simulink model "cubesat_propagation"  (R2019b)
settings: Solver=FixedStepAuto  StartTime=0.0  StopTime=5  FixedStep=dT  RelTol=1e-5
PostLoadFcn:
  | if builtin('license','test','Virtual_Reality_Toolbox')
  |     set_param([bdroot(gcs) '/Simulink 3D Animation'], 'enableVis', 'on')
  | else
  |     set_param([bdroot(gcs) '/Simulink 3D Animation'], 'enableVis', 'off')
  | end
InitFcn:
  | if strcmp(get_param([bdroot(gcs) '/Simulink 3D Animation'], 'enableVis'), 'on')
  |     if ~builtin('license','checkout','Virtual_Reality_Toolbox')
  |         error(message('aeroblks_cubesat:cubesat:licenseFailAnimTemplate'));
  |     end
  | end
model workspace (MATLAB code in the model file + MAT data in the model file):
  aeroCoeff.Cl0 = 0.000591
  aeroCoeff.Cl_beta = -0.0618
  aeroCoeff.Cl_da = -0.09917
  aeroCoeff.Cl_da_alpha = -0.08269
  aeroCoeff.Cl_dr = 0.006934
  aeroCoeff.Cl_p = -0.5045
  aeroCoeff.Cl_r = 0.1695
  aeroCoeff.Cm0 = 0.09448
  aeroCoeff.Cm_alpha = -0.6028
  aeroCoeff.Cm_alpha2 = -2.14
  aeroCoeff.Cm_beta2 = 0.6921
  aeroCoeff.Cm_de = -1.921
  aeroCoeff.Cm_df = 0.4072
  aeroCoeff.Cm_q = -15.56
  aeroCoeff.Cm_r = -0.3118
  aeroCoeff.Cn0 = -0.003117
  aeroCoeff.Cn_beta = 0.006719
  aeroCoeff.Cn_beta3 = 0.1373
  aeroCoeff.Cn_da = -0.003872
  aeroCoeff.Cn_dr = -0.08265
  aeroCoeff.Cn_p = -0.1585
  aeroCoeff.Cn_q = 0.1595
  aeroCoeff.Cn_r = -0.1112
  aeroCoeff.Cx0 = -0.03554
  aeroCoeff.Cx_alpha = 0.00292
  aeroCoeff.Cx_alpha2 = 5.459
  aeroCoeff.Cx_alpha3 = -5.162
  aeroCoeff.Cx_df = -0.09447
  aeroCoeff.Cx_df_alpha = 1.106
  aeroCoeff.Cx_dr = 0.03412
  aeroCoeff.Cx_q = -0.6748
  aeroCoeff.Cy0 = -0.002226
  aeroCoeff.Cy_beta = -0.7678
  aeroCoeff.Cy_da = -0.02956
  aeroCoeff.Cy_dr = 0.1158
  aeroCoeff.Cy_dr_alpha = 0.5238
  aeroCoeff.Cy_p = -0.124
  aeroCoeff.Cy_r = 0.3666
  aeroCoeff.Cz0 = -0.05504
  aeroCoeff.Cz_alpha = -5.578
  aeroCoeff.Cz_alpha3 = 3.442
  aeroCoeff.Cz_de = -0.398
  aeroCoeff.Cz_de_beta = -15.93
  aeroCoeff.Cz_df = -1.377
  aeroCoeff.Cz_df_alpha = -1.261
  aeroCoeff.Cz_q = -2.988
  environment.EarthRefAlt = 0
  initCond.x0 = [0 0 -2202]
  initCond.v0 = [44.54 2.714 5.836]
  initCond.euler0 = [0 0.1308996939 0]
  initCond.w0 = [0 0 0]
  inputs0.time = 0
  inputs0.signals(1).dimensions = 1
  inputs0.signals(1).values = -0.104711430294
  inputs0.signals(2).dimensions = 1
  inputs0.signals(2).values = -0.0698725229544
  inputs0.signals(3).dimensions = 1
  inputs0.signals(3).values = -0.000215042330254
  states0.time = 0
  states0.signals(1).values = [0 0 -2202]
  states0.signals(1).dimensions = 3
  states0.signals(1).label = 'CSTATE'
  states0.signals(1).blockName = 'asb6DOFAirframeTemplate/6DOF EOM/6DOF (Euler Angles)/xe,ye,ze'
  states0.signals(1).stateName = ''
  states0.signals(1).inReferencedModel = 0
  states0.signals(1).sampleTime = [0 0]
  states0.signals(2).values = [0.128665353089 0.259337659946 -0.178947917154]
  states0.signals(2).dimensions = 3
  states0.signals(2).label = 'CSTATE'
  states0.signals(2).blockName = 'asb6DOFAirframeTemplate/6DOF EOM/6DOF (Euler Angles)/Calculate DCM &
    | Euler Angles/phi
    | theta
    | psi'
  states0.signals(2).stateName = ''
  states0.signals(2).inReferencedModel = 0
  states0.signals(2).sampleTime = [0 0]
  states0.signals(3).values = [36.9119692666 8.10720863264 8.82591882596]
  states0.signals(3).dimensions = 3
  states0.signals(3).label = 'CSTATE'
  states0.signals(3).blockName = 'asb6DOFAirframeTemplate/6DOF EOM/6DOF (Euler Angles)/ub,vb,wb'
  states0.signals(3).stateName = ''
  states0.signals(3).inReferencedModel = 0
  states0.signals(3).sampleTime = [0 0]
  states0.signals(4).values = [0 0 0]
  states0.signals(4).dimensions = 3
  states0.signals(4).label = 'CSTATE'
  states0.signals(4).blockName = 'asb6DOFAirframeTemplate/6DOF EOM/6DOF (Euler Angles)/p,q,r '
  states0.signals(4).stateName = ''
  states0.signals(4).inReferencedModel = 0
  states0.signals(4).sampleTime = [0 0]
  states0.signals(5).values = [0 0]
  states0.signals(5).dimensions = 2
  states0.signals(5).label = 'CSTATE'
  states0.signals(5).blockName = 'asb6DOFAirframeTemplate/Environment Model/Dryden Wind Turbulence Model 
    | (Continuous (+q +r))/Filters on velocities/Hwgw(s)/wg_p1'
  states0.signals(5).stateName = ''
  states0.signals(5).inReferencedModel = 0
  states0.signals(5).sampleTime = [0 0]
  states0.signals(6).values = [0 0]
  states0.signals(6).dimensions = 2
  states0.signals(6).label = 'CSTATE'
  states0.signals(6).blockName = 'asb6DOFAirframeTemplate/Environment Model/Dryden Wind Turbulence Model 
    | (Continuous (+q +r))/Filters on velocities/Hwgw(s)/wg_p2'
  states0.signals(6).stateName = ''
  states0.signals(6).inReferencedModel = 0
  states0.signals(6).sampleTime = [0 0]
  states0.signals(7).values = [0 0]
  states0.signals(7).dimensions = 2
  states0.signals(7).label = 'CSTATE'
  states0.signals(7).blockName = 'asb6DOFAirframeTemplate/Environment Model/Dryden Wind Turbulence Model 
    | (Continuous (+q +r))/Filters on velocities/Hvgw(s)/vg_p1'
  states0.signals(7).stateName = ''
  states0.signals(7).inReferencedModel = 0
  states0.signals(7).sampleTime = [0 0]
  states0.signals(8).values = [0 0]
  states0.signals(8).dimensions = 2
  states0.signals(8).label = 'CSTATE'
  states0.signals(8).blockName = 'asb6DOFAirframeTemplate/Environment Model/Dryden Wind Turbulence Model 
    | (Continuous (+q +r))/Filters on velocities/Hvgw(s)/vgw_p2'
  states0.signals(8).stateName = ''
  states0.signals(8).inReferencedModel = 0
  states0.signals(8).sampleTime = [0 0]
  states0.signals(9).values = [0 0]
  states0.signals(9).dimensions = 2
  states0.signals(9).label = 'CSTATE'
  states0.signals(9).blockName = 'asb6DOFAirframeTemplate/Environment Model/Dryden Wind Turbulence Model 
    | (Continuous (+q +r))/Filters on velocities/Hugw(s)/ug_p'
  states0.signals(9).stateName = ''
  states0.signals(9).inReferencedModel = 0
  states0.signals(9).sampleTime = [0 0]
  states0.signals(10).values = [0 0]
  states0.signals(10).dimensions = 2
  states0.signals(10).label = 'CSTATE'
  states0.signals(10).blockName = 'asb6DOFAirframeTemplate/Environment Model/Dryden Wind Turbulence Model 
    | (Continuous (+q +r))/Filters on angular rates/Hrgw/rgw_p'
  states0.signals(10).stateName = ''
  states0.signals(10).inReferencedModel = 0
  states0.signals(10).sampleTime = [0 0]
  states0.signals(11).values = [0 0]
  states0.signals(11).dimensions = 2
  states0.signals(11).label = 'CSTATE'
  states0.signals(11).blockName = 'asb6DOFAirframeTemplate/Environment Model/Dryden Wind Turbulence Model 
    | (Continuous (+q +r))/Filters on angular rates/Hqgw/qgw_p'
  states0.signals(11).stateName = ''
  states0.signals(11).inReferencedModel = 0
  states0.signals(11).sampleTime = [0 0]
  states0.signals(12).values = [0 0]
  states0.signals(12).dimensions = 2
  states0.signals(12).label = 'CSTATE'
  states0.signals(12).blockName = 'asb6DOFAirframeTemplate/Environment Model/Dryden Wind Turbulence Model 
    | (Continuous (+q +r))/Filters on angular rates/Hpgw/pgw_p'
  states0.signals(12).stateName = ''
  states0.signals(12).inReferencedModel = 0
  states0.signals(12).sampleTime = [0 0]
  vehicle.Sref = 23.23
  vehicle.cbar = 1.5875
  vehicle.bref = 14.63
  vehicle.CG = [0 0 0]
  vehicle.CP = [0 0 0]
  vehicle.inertia = [5788  0  117.6; 0  6928.9  0; -117.6  0  11578.3]
  vehicle.acMass = 2288.231
  vehicle.Thrust = 2300
  vehicle.aileron_max = 0.523598775598
  vehicle.aileron_min = -0.523598775598
  vehicle.elevator_max = 0.523598775598
  vehicle.elevator_min = -0.523598775598
  vehicle.rudder_max = 1.0471975512
  vehicle.rudder_min = -1.0471975512
  other statements: initialize6DOFSkyHogg;
values from neighbouring files (symbols this model uses):
  a = (mu^(1/3))/((2*n*pi/86400)^(2/3))+0.01e5    (= 6961989.91401)    [pwsat2_setup.m]
  e = 0.0011871    [pwsat2_setup.m]
  incl = deg2rad(97.7672)    [pwsat2_setup.m]
  initEuler = [0 0 0]    [pwsat2_setup.m]
  julian = juliandate(utc)    [pwsat2_setup.m]
  RA = deg2rad(56.1804)    [pwsat2_setup.m]
  w = deg2rad(236.0402)    [pwsat2_setup.m]
undefined symbols (not defined in the file or in its folder): constraintAxes, Earth, euler0, km, pointing, pqr0, s, TA, WGS84
libraries: aerolibutil x13, aerolibconvert2 x5, sharedtransform x3, asbCubeSatBlockLib x2, simulink x2, aerolibcelestial x2, aerolib6dof2 x1, aerolibtransform2 x1, sharedutil x1, aerolibobsolete x1, vrlib x1, aerolibgravity2 x1
(part 1 of 2)
settings Model: Creator=asmialek  LastModifiedBy=asmialek
settings SolverCC: AutoInsertRateTranBlk=on  InsertRTBMode=Never (minimum delay)  MinimalZcImpactIntegration=on
settings DataIOCC: SaveFormat=Array  SaveOutput=off  SignalLogging=off  DSMLogging=off  ReturnWorkspaceOutputsName=cube
settings OptimizationCC: EnhancedBackFolding=on  StrengthReduction=on  InitFltsAndDblsToZero=on  DifferentSizesBufferReuse=on
settings DebuggingCC: WriteAfterWriteMsg=DisableAll  AlgebraicLoopMsg=none  FcnCallInpInsideContextMsg=warning  UnconnectedInputMsg=none  UnconnectedOutputMsg=none  UnconnectedLineMsg=none  UniqueDataStoreMsg=error  RootOutportRequireBusObject=none  StateNameClashWarn=warning  PregeneratedLibrarySubsystemCodeDiagnostic=none  StrictBusMsg=ErrorOnBusTreatedAsVector  SFUnexpectedBacktrackingDiag=warning  SFNoUnconditionalDefaultTransitionDiag=warning  SFExecutionAtInitializationDiag=none  ArithmeticOperatorsInVariantConditions=warning
settings ModelReferenceCC: PropagateSignalLabelsOutOfModel=off
settings SFSimCC: SimUseLocalCustomCode=off  CustomCodeUndefinedFunction=UseInterfaceOnly
settings RTWCC: RTWUseLocalCustomCode=off
settings CodeAppCC: StateflowObjectComments=on

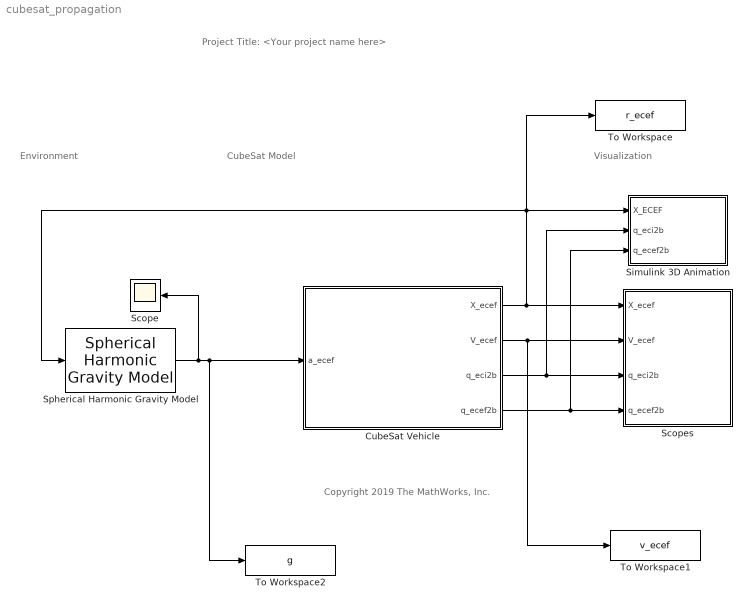
== system cubesat_propagation ==
  note: Project Title: <Your project name here>
  note: Copyright 2019 The MathWorks, Inc.
  note: Visualization
  note: Environment
  note: CubeSat Model
  CubeSat Vehicle : Subsystem  AncestorBlock=asbCubeSatBlockLib/CubeSat Vehicle  BlockKeywords=__PRM__SERIALIZED__DATA__:cube sat,cube sat vehicle,satellite,nanosat,nano sat,nanosatellite,nano satellite,pico sat,picosat,pico satellite,picosatellite,orbit propagator,orbit propagation,orbital propagator,orbital dynamics,astrodynamics,astro dynamics,spacecraft,space craft,space vehicle,spaceflight,space flight,low Earth orbit,low-Earth orbit,attitude control,kepler,keplerian elements,orbital elements,ECI,ECEF,Earth orientation parameters  mask(CubeSat Vehicle){sim_t0=julian, method=Keplerian Orbital Elements, epoch=2451545, a=a, ecc=e, incl=rad2deg(incl), omega=rad2deg(RA), argp=rad2deg(w), nu=rad2deg(TA), truelon=0, arglat=0, lonper=0, r_eci=[0 0 0], v_eci=[0 0 0], r_ecef=[0 0 0], v_ecef=[0 0 0], lla=[0 0 0], v_ned=[0 0 0], euler=initEuler, pqr=[0 0 0], pointingMode=Standby (Off), firstAlignExt=Dialog, firstAlign=[0 0 1], secondAlignExt=Dialog, secondAlign=[0 1 0], constraintCoord=ECI Axes, firstRefExt=Dialog, firstRef=[1 0 0], secondRefExt=Dialog, secondRef=[0 0 1], eopExt=Dialog, dAT=37, dUT1=-0.1193, pm=[0.2141e-4 0.6930e-4], dCIP=[0.1014e-6  -0.0681e-6], lod=0, missionRTSource=Dialog, missionRT=6*60*60, missionGS=[42, -71], missionTOICheck=on, missionTOI=[], missionEta=55, missionName=}
      mask prompts: sim_t0 "aeroblks_cubesat:cubesat:StartDate"; method "aeroblks_cubesat:cubesat:InputMethod"; epoch "aeroblks_cubesat:cubesat:ECIEpoch"; a "aeroblks_cubesat:cubesat:SemiMajorAxis"; ecc "aeroblks_cubesat:cubesat:Eccentricity"; incl "aeroblks_cubesat:cubesat:Inclination"; omega "aeroblks_cubesat:cubesat:RAAN"; argp "aeroblks_cubesat:cubesat:ArgP"; nu "aeroblks_cubesat:cubesat:TrueAnomaly"; truelon "aeroblks_cubesat:cubesat:TrueLon"; arglat "aeroblks_cubesat:cubesat:ArgLat"; lonper "aeroblks_cubesat:cubesat:LonPer"; r_eci "aeroblks_cubesat:cubesat:ECIPos"; v_eci "aeroblks_cubesat:cubesat:ECIVel"; r_ecef "aeroblks_cubesat:cubesat:ECEFPos"; v_ecef "aeroblks_cubesat:cubesat:ECEFVel"; lla "aeroblks_cubesat:cubesat:LLA"; v_ned "aeroblks_cubesat:cubesat:NEDVel"; euler "aeroblks_cubesat:cubesat:Euler"; pqr "aeroblks_cubesat:cubesat:BodyAngRates"; pointingMode "aeroblks_cubesat:cubesat:PointingMode"; constraintCoord "aeroblks_cubesat:cubesat:ConstaintCoord"; eopExt "aeroblks_cubesat:cubesat:EOPPulldown"; dAT "aeroblks_cubesat:cubesat:dTAI"; dUT1 "aeroblks_cubesat:cubesat:DUT1"; pm "aeroblks_cubesat:cubesat:DPolar"; dCIP "aeroblks_cubesat:cubesat:DCIP"; lod "aeroblks_cubesat:cubesat:DLOD"; missionRTSource "aeroblks_cubesat:cubesat:MissRunTimeSource"; missionRT "aeroblks_cubesat:cubesat:MissRunTime"; missionGS "aeroblks_cubesat:cubesat:MissGS"; missionTOICheck "aeroblks_cubesat:cubesat:MissTOICheckbox"; missionTOI "aeroblks_cubesat:cubesat:MissTOI"; missionEta "aeroblks_cubesat:cubesat:MissEta"; missionName "aeroblks_cubesat:cubesat:MissFileName"
      mask help: aeroblks_cubesat:cubesat:CubeSatBlockDesc
      mask init:
      | [lla0, uvw0, euler0, pqr0, thGAST0, ports, constraintAxes, pointing]  = cubesatBlockCallback(...
      |     gcb, 'init', method, sim_t0, epoch, a, ecc, incl, omega,...
      |     argp, nu, truelon, arglat, lonper,r_eci, v_eci, r_ecef, v_ecef,...
      |     lla, v_ned, euler, pqr, dAT, dUT1, pm, dCIP, lod);
      settings: AttributesFormatString=%<pointingMode>
      mask Help: helpview(fullfile(docroot,'aeroblks','aeroblks.map'),'cubesatvehicle')
      mask TypeOptions method: aeroblks_cubesat:cubesat:InputKeplerian | aeroblks_cubesat:cubesat:InputECI | aeroblks_cubesat:cubesat:InputECEF | aeroblks_cubesat:cubesat:InputLLANED
      mask Callback method: cubesatBlockCallback(gcb, 'method');
      mask Callback ecc: cubesatBlockCallback(gcb, 'circ');
      mask Callback incl: cubesatBlockCallback(gcb, 'circ');
      mask TypeOptions pointingMode: aeroblks_cubesat:cubesat:PointingNadir | aeroblks_cubesat:cubesat:PointingSun | aeroblks_cubesat:cubesat:PointingCustom | aeroblks_cubesat:cubesat:PointingOff
      mask Callback pointingMode: cubesatBlockCallback(gcb, 'pointing');
      mask TypeOptions firstAlignExt: aeroblks_cubesat:cubesat:SourceDialog | aeroblks_cubesat:cubesat:SourcePort
      mask Callback firstAlignExt: cubesatBlockCallback(gcb, 'pointingExt');
      mask TypeOptions secondAlignExt: aeroblks_cubesat:cubesat:SourceDialog | aeroblks_cubesat:cubesat:SourcePort
      mask Callback secondAlignExt: cubesatBlockCallback(gcb, 'pointingExt');
      mask TypeOptions constraintCoord: aeroblks_cubesat:cubesat:ConstaintECI | aeroblks_cubesat:cubesat:ConstaintECEF | aeroblks_cubesat:cubesat:ConstaintNED | aeroblks_cubesat:cubesat:ConstaintBody
      mask TypeOptions firstRefExt: aeroblks_cubesat:cubesat:SourceDialog | aeroblks_cubesat:cubesat:SourcePort
      mask Callback firstRefExt: cubesatBlockCallback(gcb, 'pointingExt');
      mask TypeOptions secondRefExt: aeroblks_cubesat:cubesat:SourceDialog | aeroblks_cubesat:cubesat:SourcePort
      mask Callback secondRefExt: cubesatBlockCallback(gcb, 'pointingExt');
      mask TypeOptions eopExt: aeroblks_cubesat:cubesat:SourceDialog | aeroblks_cubesat:cubesat:SourcePort
      mask TypeOptions missionRTSource: Dialog | Model StopTime
      mask Callback missionRTSource: cubesatBlockCallback(gcb, 'mission');
      mask Callback missionTOICheck: cubesatBlockCallback(gcb, 'mission');
      mask DialogControl sim_t0 Prompt: Start date [Julian date]:
      mask DialogControl sim_t0 Tooltip: aeroblks_cubesat:cubesat:StartDateTT
      mask DialogControl orbit Prompt: aeroblks_cubesat:cubesat:OrbitTab
      mask DialogControl method Prompt: Input method:
      mask DialogControl method Tooltip: aeroblks_cubesat:cubesat:InputMethodTT
      mask DialogControl epoch Prompt: Epoch of ECI frame [Julian date]:
      mask DialogControl epoch Tooltip: aeroblks_cubesat:cubesat:ECIEpochTT
      mask DialogControl a Prompt: Semi-major axis [m]:
      mask DialogControl a Tooltip: aeroblks_cubesat:cubesat:SemiMajorAxisTT
      mask DialogControl ecc Prompt: Eccentricity:
      mask DialogControl ecc Tooltip: aeroblks_cubesat:cubesat:EccentricityTT
      mask DialogControl incl Prompt: Inclination [deg]:
      mask DialogControl incl Tooltip: aeroblks_cubesat:cubesat:InclinationTT
      mask DialogControl omega Prompt: Right ascension of the ascending node [deg]:
      mask DialogControl omega Tooltip: aeroblks_cubesat:cubesat:RAANTT
      mask DialogControl argp Prompt: Argument of periapsis [deg]:
      mask DialogControl argp Tooltip: aeroblks_cubesat:cubesat:ArgPTT
      mask DialogControl nu Prompt: True anomaly [deg]:
      mask DialogControl nu Tooltip: aeroblks_cubesat:cubesat:TrueAnomalyTT
      mask DialogControl truelon Prompt: True longitude [deg] (circular equatorial):
      mask DialogControl truelon Tooltip: aeroblks_cubesat:cubesat:TrueLonTT
      mask DialogControl arglat Prompt: Argument of latitude [deg] (circular inclined):
      mask DialogControl arglat Tooltip: aeroblks_cubesat:cubesat:ArgLatTT
      mask DialogControl lonper Prompt: Longitude of periapsis [deg] (elliptical equatorial):
      mask DialogControl lonper Tooltip: aeroblks_cubesat:cubesat:LonPerTT
      mask DialogControl r_eci Prompt: ECI position vector [m]:
      mask DialogControl r_eci Tooltip: aeroblks_cubesat:cubesat:ECIPosTT
      mask DialogControl v_eci Prompt: ECI velocity vector [m/s]:
      mask DialogControl v_eci Tooltip: aeroblks_cubesat:cubesat:ECIVelTT
      mask DialogControl r_ecef Prompt: ECEF position vector [m]:
      mask DialogControl r_ecef Tooltip: aeroblks_cubesat:cubesat:ECEFPosTT
      mask DialogControl v_ecef Prompt: ECEF velocity vector [m/s]:
      mask DialogControl v_ecef Tooltip: aeroblks_cubesat:cubesat:ECEFVelTT
      mask DialogControl lla Prompt: Geodetic latitude, longitude, altitude [deg, deg, m]:
      mask DialogControl lla Tooltip: aeroblks_cubesat:cubesat:LLATT
      mask DialogControl v_ned Prompt: NED velocity vector [m/s]:
      mask DialogControl v_ned Tooltip: aeroblks_cubesat:cubesat:NEDVelTT
      mask DialogControl Container12 Prompt: aeroblks_cubesat:cubesat:AttitudeTab
      mask DialogControl euler Prompt: <html>Initial Euler angles (roll, pitch, yaw) [deg]:</html>
      mask DialogControl euler Tooltip: aeroblks_cubesat:cubesat:EulerTT
      mask DialogControl pqr Prompt: Initial body angular rates [deg/s]:
      mask DialogControl pqr Tooltip: aeroblks_cubesat:cubesat:BodyAngRatesTT
      mask DialogControl Container8 Prompt: aeroblks_cubesat:cubesat:AttitudeControlArea
      mask DialogControl pointingMode Prompt: Pointing mode:
      mask DialogControl pointingMode Tooltip: aeroblks_cubesat:cubesat:PointingModeTT
      mask DialogControl firstAlignText Prompt: aeroblks_cubesat:cubesat:PrimAlign
      mask DialogControl firstAlignExt Tooltip: aeroblks_cubesat:cubesat:PrimAlignPulldownTT
      mask DialogControl firstAlign Tooltip: aeroblks_cubesat:cubesat:PrimAlignDialogTT
      mask DialogControl secondAligntext Prompt: aeroblks_cubesat:cubesat:SecAlign
      mask DialogControl secondAlignExt Tooltip: aeroblks_cubesat:cubesat:SecAlignPulldownTT
      mask DialogControl secondAlign Tooltip: aeroblks_cubesat:cubesat:SecAlignDialogTT
      mask DialogControl constraintCoord Prompt: Constraint coordinate system:
      mask DialogControl constraintCoord Tooltip: aeroblks_cubesat:cubesat:ConstaintCoordTT
      mask DialogControl firstRefText Prompt: aeroblks_cubesat:cubesat:PrimConstraint
      mask DialogControl firstRefExt Tooltip: aeroblks_cubesat:cubesat:PrimConstraintPulldownTT
      mask DialogControl firstRef Tooltip: aeroblks_cubesat:cubesat:PrimConstraintDialogTT
      mask DialogControl secondRefText Prompt: aeroblks_cubesat:cubesat:SecConstraint
      mask DialogControl secondRefExt Tooltip: aeroblks_cubesat:cubesat:SecConstraintPulldownTT
      mask DialogControl secondRef Tooltip: aeroblks_cubesat:cubesat:SecConstraintDialogTT
      mask DialogControl epTab Prompt: Earth Orientation Parameters
      mask DialogControl eopExt Prompt: hidden
      mask DialogControl dAT Prompt: Difference between TAI and UTC [sec]:
      mask DialogControl dAT Tooltip: aeroblks_cubesat:cubesat:dTAITT
      mask DialogControl dUT1 Prompt: Difference between UTC and UT1 [sec]:
      mask DialogControl dUT1 Tooltip: aeroblks_cubesat:cubesat:DUT1TT
      mask DialogControl pm Prompt: Polar displacement [deg deg]:
      mask DialogControl pm Tooltip: aeroblks_cubesat:cubesat:DPolarTT
      mask DialogControl dCIP Prompt: CIP adjustment [deg deg]:
      mask DialogControl dCIP Tooltip: aeroblks_cubesat:cubesat:DCIPTT
      mask DialogControl lod Prompt: Excess length of day [sec]:
      mask DialogControl lod Tooltip: aeroblks_cubesat:cubesat:DLODTT
      mask DialogControl Container11 Prompt: Mission Analysis
      mask DialogControl missionText Prompt: aeroblks_cubesat:cubesat:MissText
      mask DialogControl missionRTSource Prompt: Analysis run time source:
      mask DialogControl missionRTSource Tooltip: aeroblks_cubesat:cubesat:MissRunTimeSourceTT
      mask DialogControl missionRT Prompt: Run time [sec]:
      mask DialogControl missionRT Tooltip: aeroblks_cubesat:cubesat:MissRunTimeTT
      mask DialogControl missionGS Prompt: Ground station geodetic latitude, longitude [deg, deg]:
      mask DialogControl missionGS Tooltip: aeroblks_cubesat:cubesat:MissGSTT
      mask DialogControl Container10 Prompt: aeroblks_cubesat:cubesat:MissTOITab
      mask DialogControl missionTOICheck Prompt: Run TOI analysis
      mask DialogControl missionTOICheck Tooltip: aeroblks_cubesat:cubesat:MissTOICheckboxTT
      mask DialogControl missionTOI Prompt: Time of interest [Julian date]:
      mask DialogControl missionTOI Tooltip: aeroblks_cubesat:cubesat:MissTOITT
      mask DialogControl missionEta Prompt: Camera field-of-view (FOV) half angle [deg]:
      mask DialogControl missionEta Tooltip: aeroblks_cubesat:cubesat:MissEtaTT
      mask DialogControl missionName Prompt: Live script file name:
      mask DialogControl missionName Tooltip: aeroblks_cubesat:cubesat:MissFileNameTT
      mask DialogControl missionOpen Prompt: aeroblks_cubesat:cubesat:MissCreate
      mask DialogControl missionOpen Tooltip: aeroblks_cubesat:cubesat:MissCreateTT
      mask DialogControl missionOpen Callback:
      | maskvals = get_param(gcb,'MaskValues');
      | generateMissionReport(gcb, maskvals{43},...
      |     maskvals{39}, 'RuntimeSource', maskvals{37},...
      |     'Runtime', maskvals{38}, 'EnableTOI',...
      |     maskvals{40}, 'TOI', maskvals{41}, 'Eta',...
      |     maskvals{42})
      | clear maskvals
      mask Display:
      | port_label(ports(1).type,ports(1).port,ports(1).txt,'texmode','on');
      | port_label(ports(2).type,ports(2).port,ports(2).txt,'texmode','on');
      | port_label(ports(3).type,ports(3).port,ports(3).txt,'texmode','on');
      | port_label(ports(4).type,ports(4).port,ports(4).txt,'texmode','on');
      | port_label(ports(5).type,ports(5).port,ports(5).txt,'texmode','on');
      | port_label(ports(6).type,ports(6).port,ports(6).txt,'texmode','on');
      | port_label(ports(7).type,ports(7).port,ports(7).txt,'texmode','on');
      | port_label(ports(8).type,ports(8).port,ports(8).txt,'texmode','on');
      | port_label(ports(9).type,ports(9).port,ports(9).txt,'texmode','on');
  Scope : Scope
  Scopes : Subsystem  VariantControl=visOff
  Simulink 3D Animation : Subsystem  mask(Set Animation Properties){enableVis=on, startDate=2458488, visSampleTime=5, cubesatSize=2e5, showAntenna=on, antennaHeight=1e6, antennaHalfAngle=25}
      mask prompts: enableVis "aeroblks_cubesat:cubesat:AnimEnableVis"; startDate "aeroblks_cubesat:cubesat:StartDate"; visSampleTime "aeroblks_cubesat:cubesat:AnimSampleTime"; cubesatSize "aeroblks_cubesat:cubesat:MdlSize"; showAntenna "aeroblks_cubesat:cubesat:ShowCone"; antennaHeight "aeroblks_cubesat:cubesat:ConeHeight"; antennaHalfAngle "aeroblks_cubesat:cubesat:ConeAngle"
      mask help: aeroblks_cubesat:cubesat:VisBlockDesc
      settings: OpenFcn=|
      | if ~builtin('license','test','virtual_reality_toolbox')
      |     set_param(gcb, 'enableVis', 'off');
      | end
      | open_system(gcb,'mask');
      mask Callback enableVis:
      | if strcmp(get_param(gcb,'enableVis'), 'on')
      |     [licAvail, ~] = builtin('license','checkout','Virtual_Reality_Toolbox');
      |     if licAvail
      |         enable = repmat({'on'},7,1);
      |         set_param(gcb, 'Commented', 'off');
      |     else
      |         enable = repmat({'off'},7,1);
      |         set_param(gcb, 'Commented', 'on');
      |         set_param(gcb,'enableVis', 'off');
      |     end
      |     clear licAvail
      | else
      |     enable = repmat({'off'},7,1);
      |     set_param(gcb, 'Commented', 'on');
      | end
      | enable{1} = 'on';
      | set_param(gcb,'MaskEnables', enable);
      | clear enable
      mask Callback showAntenna:
      | if strcmp(get_param(gcb, 'enableVis'), 'on')
      |     enable = get_param(gcb,'MaskEnables');
      |     if strcmp(get_param(gcb, 'showAntenna'), 'off')
      |         enable(6:7) = {'off'};
      |     else
      |         enable(6:7) = {'on'};
      |     end
      |     set_param(gcb,'MaskEnables', enable);
      |     clear enable
      | end
      mask DialogControl enableVis Prompt: Enable visualization with Simulink 3D Animation
      mask DialogControl vrOpenBtn Prompt: aeroblks_cubesat:cubesat:AnimOpenBtn
      mask DialogControl vrOpenBtn Callback:
      | if builtin('license','checkout','Virtual_Reality_Toolbox')
      |     vrmfunc('FnOpen',getSimulinkBlockHandle([gcb '/VR Sink']));
      | end
      mask DialogControl startDate Prompt: Start date [Julian date]:
      mask DialogControl startDate Tooltip: aeroblks_cubesat:cubesat:StartDateTT
      mask DialogControl visSampleTime Prompt: Animation refresh rate:
      mask DialogControl visSampleTime Tooltip: aeroblks_cubesat:cubesat:AnimSampleTimeTT
      mask DialogControl cubesatSize Prompt: CubeSat display size [m]:
      mask DialogControl cubesatSize Tooltip: aeroblks_cubesat:cubesat:MdlSizeTT
      mask DialogControl Container3 Prompt: aeroblks_cubesat:cubesat:AntennaPropArea
      mask DialogControl showAntenna Prompt: Show antenna cone in animation
      mask DialogControl showAntenna Tooltip: aeroblks_cubesat:cubesat:ShowConeTT
      mask DialogControl antennaHeight Prompt: Antenna cone height [m]:
      mask DialogControl antennaHeight Tooltip: aeroblks_cubesat:cubesat:ConeHeightTT
      mask DialogControl antennaHalfAngle Prompt: Antenna cone half angle [deg]:
      mask DialogControl antennaHalfAngle Tooltip: aeroblks_cubesat:cubesat:ConeAngleTT
      mask Display:
      | port_label('input', 1, 'X_{ECEF}','texmode','on')
      | port_label('input', 2, 'q_{ECI2Body}','texmode','on')
      | port_label('input', 3, 'X_{ECEF2Body}','texmode','on')
  Spherical Harmonic Gravity Model : aerolibgravity2/Spherical Harmonic Gravity Model  RequirementInfo={} %GIDa_bac5afc4_2ad9_46dd_a955_1e359e941ebd  units=Metric (MKS)  degree=20  action=Warning  ptype=EGM2008  datafile='aerogmm2b.mat'
      settings: SourceProductName=Aerospace Blockset  SourceProductBaseCode=AE
  To Workspace : ToWorkspace  VariableName=r_ecef  SampleTime=-1
  To Workspace1 : ToWorkspace  VariableName=v_ecef  SaveFormat=Timeseries  SampleTime=-1
  To Workspace2 : ToWorkspace  VariableName=g  SaveFormat=Timeseries  SampleTime=-1
  wires:
  Spherical Harmonic Gravity Model/1 -> To Workspace2/1, CubeSat Vehicle/1(a_ecef), Scope/1
  CubeSat Vehicle/1(X_ecef) -> Scopes/1(X_ecef), To Workspace/1, Spherical Harmonic Gravity Model/1, Simulink 3D Animation/1(X_ECEF)
  CubeSat Vehicle/3(q_eci2b) -> Simulink 3D Animation/2(q_eci2b), Scopes/3(q_eci2b)
  CubeSat Vehicle/2(V_ecef) -> To Workspace1/1, Scopes/2(V_ecef)
  CubeSat Vehicle/4(q_ecef2b) -> Simulink 3D Animation/3(q_ecef2b), Scopes/4(q_ecef2b)

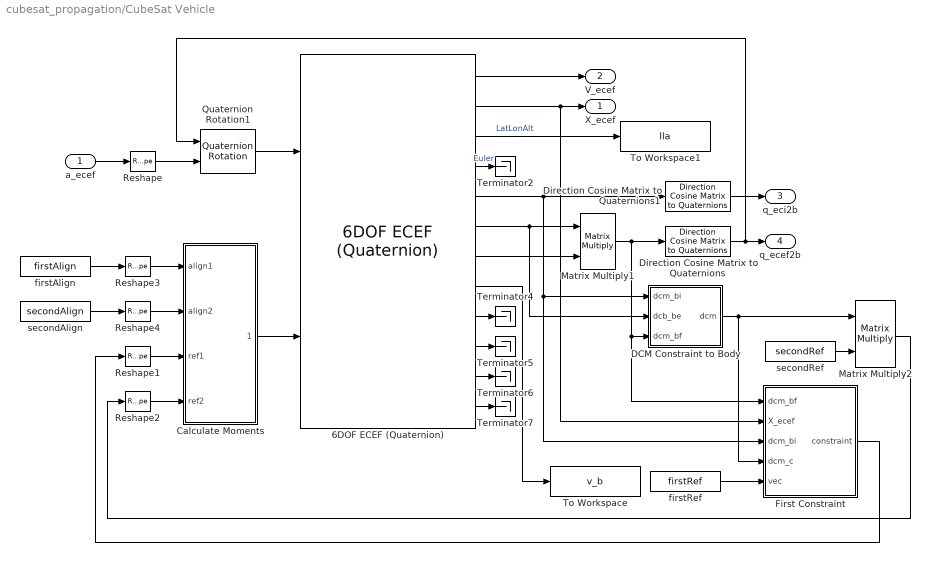
== system cubesat_propagation/CubeSat Vehicle ==
  a_ecef : Inport
  6DOF ECEF (Quaternion) : aerolib6dof2/6DOF ECEF (Quaternion)  units=Metric (MKS)  mtype=Fixed  xg_0=lla0  Vm_0=uvw0  eul_0=euler0*pi/180  pm_0=pqr0*pi/180  mass_0=1  mass_e=0.5  mass_f=2.0  inertia=eye(3)  inertia_e=eye(3)  inertia_f=2*eye(3)  vre_flag=on  abi_flag=off  ptype=Earth (WGS84)  R=6378137  F=1/298.257223563  w_E=7292115e-11  angle_in=Internal  LG0=thGAST0  quat_statename=''  pm_statename=''  Vm_statename=''  posECEF_statename=''  posECI_statename=''  LG_statename=''  mass_statename=''
      settings: SourceProductName=Aerospace Blockset  SourceProductBaseCode=AE
  Calculate Moments : Subsystem
  DCM Constraint to Body : Subsystem
  Direction Cosine Matrix to Quaternions : sharedtransform/Direction Cosine Matrix  to Quaternions  aMode=0  action=None  tolerance=eps(2)
      settings: SourceProductName=Aerospace Blockset  SourceProductBaseCode=AE
  Direction Cosine Matrix to Quaternions1 : sharedtransform/Direction Cosine Matrix  to Quaternions  aMode=0  action=None  tolerance=eps(2)
      settings: SourceProductName=Aerospace Blockset  SourceProductBaseCode=AE
  First Constraint : Subsystem
  Matrix Multiply1 : Product  Multiplication=Matrix(*)
  Matrix Multiply2 : Product  Multiplication=Matrix(*)
  Quaternion Rotation1 : aerolibutil/Quaternion Rotation
  Reshape{,1..4} (5 alike) : Reshape
  Terminator{2,4..7} (5 alike) : Terminator
      Terminator2 settings: RequirementInfo={} %GIDa_8aaf45eb_8aca_43ab_8e8c_9139146fa2e6
      Terminator4 settings: RequirementInfo={} %GIDa_0354634f_ef6c_4a1d_80d4_86622fb9180e
      Terminator5 settings: RequirementInfo={} %GIDa_d29024c9_5e50_4e5d_bd38_ac70a5e5677e
      Terminator6 settings: RequirementInfo={} %GIDa_dae0eb2d_ace9_4114_87c0_2e7cb53e5ae5
      Terminator7 settings: RequirementInfo={} %GIDa_0bbe6eab_2da4_46ff_b2f7_37ea3444068f
  To Workspace : ToWorkspace  VariableName=v_b  SampleTime=-1
  To Workspace1 : ToWorkspace  VariableName=lla  SampleTime=-1
  firstAlign : Constant  Value=firstAlign  OutDataTypeStr=Inherit: Inherit via back propagation
  firstRef : Constant  Value=firstRef  OutDataTypeStr=Inherit: Inherit via back propagation
  secondAlign : Constant  Value=secondAlign  OutDataTypeStr=Inherit: Inherit via back propagation
  secondRef : Constant  Value=secondRef  OutDataTypeStr=Inherit: Inherit via back propagation
  X_ecef : Outport  VectorParamsAs1DForOutWhenUnconnected=off
  V_ecef : Outport  Port=2  VectorParamsAs1DForOutWhenUnconnected=off
  q_eci2b : Outport  Port=3  VectorParamsAs1DForOutWhenUnconnected=off
  q_ecef2b : Outport  Port=4  VectorParamsAs1DForOutWhenUnconnected=off
  wires:
  Reshape3/1 -> Calculate Moments/1(align1)
  First Constraint/1(constraint) -> Reshape1/1
  DCM Constraint to Body/1(dcm) -> First Constraint/4(dcm_c), Matrix Multiply2/1
  secondRef/1 -> Matrix Multiply2/2
  Reshape4/1 -> Calculate Moments/2(align2)
  firstRef/1 -> First Constraint/5(vec)
  Matrix Multiply2/1 -> Reshape2/1
  6DOF ECEF (Quaternion)/3 -> To Workspace1/1  "LatLonAlt"
  firstAlign/1 -> Reshape3/1
  Reshape2/1 -> Calculate Moments/4(ref2)
  secondAlign/1 -> Reshape4/1
  a_ecef/1 -> Reshape/1
  6DOF ECEF (Quaternion)/6 -> DCM Constraint to Body/2(dcb_be), Matrix Multiply1/1
  6DOF ECEF (Quaternion)/11 -> Terminator6/1
  Quaternion Rotation1/1 -> 6DOF ECEF (Quaternion)/1
  6DOF ECEF (Quaternion)/2 -> X_ecef/1, First Constraint/2(X_ecef)
  6DOF ECEF (Quaternion)/7 -> Matrix Multiply1/2
  6DOF ECEF (Quaternion)/5 -> DCM Constraint to Body/1(dcm_bi), First Constraint/3(dcm_bi), Direction Cosine Matrix to Quaternions1/1
  Direction Cosine Matrix to Quaternions1/1 -> q_eci2b/1
  Matrix Multiply1/1 -> Direction Cosine Matrix to Quaternions/1, DCM Constraint to Body/3(dcm_bf), First Constraint/1(dcm_bf)
  Direction Cosine Matrix to Quaternions/1 -> Quaternion Rotation1/1, q_ecef2b/1
  Calculate Moments/1(Moments) -> 6DOF ECEF (Quaternion)/2
  6DOF ECEF (Quaternion)/9 -> Terminator4/1
  Reshape1/1 -> Calculate Moments/3(ref1)
  Reshape/1 -> Quaternion Rotation1/2
  6DOF ECEF (Quaternion)/12 -> Terminator7/1
  6DOF ECEF (Quaternion)/1 -> V_ecef/1
  6DOF ECEF (Quaternion)/10 -> Terminator5/1
  6DOF ECEF (Quaternion)/4 -> Terminator2/1  "Euler"
  6DOF ECEF (Quaternion)/8 -> To Workspace/1

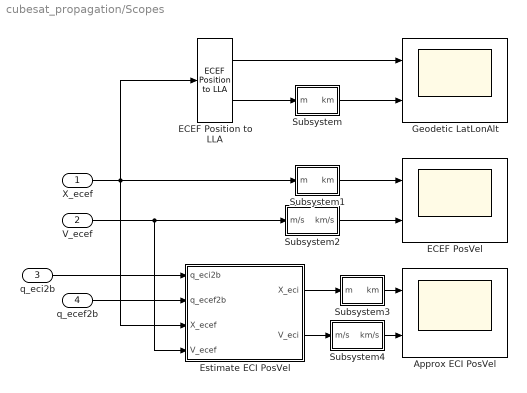
== system cubesat_propagation/Scopes ==
  X_ecef : Inport
  V_ecef : Inport  Port=2
  q_eci2b : Inport  Port=3
  q_ecef2b : Inport  Port=4
  Approx ECI PosVel : Scope  NumInputPorts=2
  ECEF PosVel : Scope  NumInputPorts=2
  ECEF Position to LLA : aerolibtransform2/ECEF Position to LLA  units=Metric (MKS)  ptype=Earth (WGS84)  F=1/298.257223563  R=6378137
      settings: SourceProductName=Aerospace Blockset  SourceProductBaseCode=AE
  Estimate ECI PosVel : Subsystem
  Geodetic LatLonAlt : Scope  NumInputPorts=2
  Subsystem : Subsystem
  Subsystem1 : Subsystem
  Subsystem2 : Subsystem
  Subsystem3 : Subsystem
  Subsystem4 : Subsystem
  wires:
  V_ecef/1 -> Subsystem2/1(m/s), Estimate ECI PosVel/4(V_ecef)
  X_ecef/1 -> ECEF Position to LLA/1, Subsystem1/1(m), Estimate ECI PosVel/3(X_ecef)
  q_ecef2b/1 -> Estimate ECI PosVel/2(q_ecef2b)
  q_eci2b/1 -> Estimate ECI PosVel/1(q_eci2b)
  Estimate ECI PosVel/2(V_eci) -> Subsystem4/1(m/s)
  Estimate ECI PosVel/1(X_eci) -> Subsystem3/1(m)
  ECEF Position to LLA/1 -> Geodetic LatLonAlt/1
  ECEF Position to LLA/2 -> Subsystem/1(m)
  Subsystem/1(km) -> Geodetic LatLonAlt/2
  Subsystem1/1(km) -> ECEF PosVel/1
  Subsystem2/1(km/s) -> ECEF PosVel/2
  Subsystem3/1(km) -> Approx ECI PosVel/1
  Subsystem4/1(km/s) -> Approx ECI PosVel/2

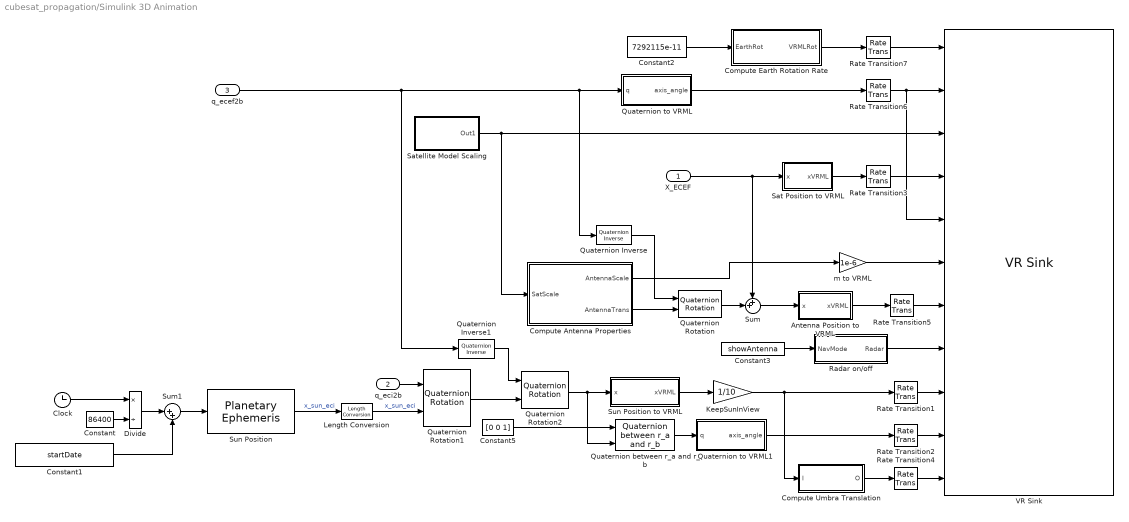
== system cubesat_propagation/Simulink 3D Animation ==
  X_ECEF : Inport
  q_eci2b : Inport  Port=2
  q_ecef2b : Inport  Port=3
  Antenna Position to VRML : Subsystem
  Clock : Clock
  Compute Antenna Properties : Subsystem
  Compute Earth Rotation Rate : Subsystem
  Compute Umbra Translation : Subsystem
  Constant : Constant  Value=86400
  Constant1 : Constant  RequirementInfo={} %GIDa_d3dce1ea_7a4c_4489_9b49_860fce94c68a  Value=startDate  SampleTime=visSampleTime
  Constant2 : Constant  RequirementInfo={} %GIDa_a027479b_4c7b_4f1d_b86b_1fc869131b24  Value=7292115e-11
  Constant3 : Constant  Value=showAntenna
  Constant5 : Constant  Value=[0 0 1]
  Divide : Product  Inputs=*/
  KeepSunInView : Gain  Gain=1/10
  Length Conversion : aerolibconvert2/Length Conversion  IU=km  OU=m
  Quaternion Inverse : aerolibutil/Quaternion Inverse
      settings: SourceProductName=Aerospace Blockset
  Quaternion Inverse1 : aerolibutil/Quaternion Inverse
      settings: SourceProductName=Aerospace Blockset
  Quaternion Rotation : aerolibutil/Quaternion Rotation
  Quaternion Rotation1 : aerolibutil/Quaternion Rotation
  Quaternion Rotation2 : aerolibutil/Quaternion Rotation
  Quaternion between r_a and r_b : asbCubeSatBlockLib/Axes Transformations/Attitude Conversion/Quaternion between r_a and r_b  SystemSampleTime=-1  Latency=0  AutoFrameSizeCalculation=off
      settings: SourceProductName=Aerospace Blockset CubeSat Simulation Library  SourceProductBaseCode=AERO_CUBESAT
  Quaternion to VRML : Subsystem
  Quaternion to VRML1 : Subsystem
  Radar on/off : Subsystem
  Rate Transition{1..7} (7 alike) : RateTransition
  Sat Position to VRML : Subsystem
  Satellite Model Scaling : Subsystem
  Sum : Sum  Inputs=++|
  Sum1 : Sum  Inputs=|++
  Sun Position : aerolibcelestial/Planetary Ephemeris  kmflag=km,km/s  epochflag=Julian date  de=DE421  nCenter=Earth  nTarget=Sun  errorflag=Error  velflag=off
      settings: SourceProductName=Aerospace Blockset  SourceProductBaseCode=AE
  Sun Position to VRML : Subsystem
  VR Sink : vrlib/VR Sink  InstantiateOnLoad=on  SampleTime=visSampleTime  ViewEnable=on  RemoteChange=off  RemoteView=off  FieldsWritten=Earth.rotation.4.1.1.double#Satellite.rotation.4.1.1.double#Satellite.scale.3.1.1.double#Satellite.translation.3.1.1.double#AntennaCone.rotation.4.1.1.double#AntennaCone.scale.3.1.1.double#AntennaCone.translation.3.1.1.double#AntennaMaterial.transparency.1.1.1.double#Sun.translation.3.1.1.double#Umbra.rotation.4.1.1.double#Umbra.translation.3.1.1.double  WorldFileName=cubesatAnim.wrl  WorldDescription=CubeSat Orbit Animation  AutoView=on  VideoDimensions=[]  AllowVariableSize=off
      settings: SourceProductName=Simulink
  m to VRML : Gain  Gain=1e-6
  wires:
  Quaternion to VRML1/1(axis_angle) -> Rate Transition2/1
  Quaternion between r_a and r_b/1 -> Quaternion to VRML1/1(q)
  Constant2/1 -> Compute Earth Rotation Rate/1(EarthRot)
  Compute Antenna Properties/1(AntennaScale) -> m to VRML/1
  Quaternion to VRML/1(axis_angle) -> Rate Transition6/1
  Compute Umbra Translation/1(O) -> Rate Transition4/1
  q_eci2b/1 -> Quaternion Rotation1/1
  Quaternion Rotation2/1 -> Sun Position to VRML/1(x), Quaternion between r_a and r_b/2
  Constant5/1 -> Quaternion between r_a and r_b/1
  KeepSunInView/1 -> Compute Umbra Translation/1(I), Rate Transition1/1
  Sun Position to VRML/1(xVRML) -> KeepSunInView/1
  Sat Position to VRML/1(xVRML) -> Rate Transition3/1
  Compute Antenna Properties/2(AntennaTrans) -> Quaternion Rotation/2
  Satellite Model Scaling/1(Out1) -> VR Sink/3, Compute Antenna Properties/1(SatScale)
  Constant3/1 -> Radar on/off/1(NavMode)
  q_ecef2b/1 -> Quaternion Inverse/1, Quaternion to VRML/1(q), Quaternion Inverse1/1
  Quaternion Rotation1/1 -> Quaternion Rotation2/2
  Compute Earth Rotation Rate/1(VRMLRot) -> Rate Transition7/1
  Antenna Position to VRML/1(xVRML) -> Rate Transition5/1
  Quaternion Inverse/1 -> Quaternion Rotation/1
  X_ECEF/1 -> Sat Position to VRML/1(x), Sum/1
  Quaternion Rotation/1 -> Sum/2
  Sum/1 -> Antenna Position to VRML/1(x)
  Quaternion Inverse1/1 -> Quaternion Rotation2/1
  Rate Transition4/1 -> VR Sink/11
  Rate Transition2/1 -> VR Sink/10
  Rate Transition1/1 -> VR Sink/9
  Rate Transition5/1 -> VR Sink/7
  m to VRML/1 -> VR Sink/6
  Rate Transition3/1 -> VR Sink/4
  Rate Transition7/1 -> VR Sink/1
  Rate Transition6/1 -> VR Sink/5, VR Sink/2
  Constant1/1 -> Sum1/2
  Divide/1 -> Sum1/1
  Constant/1 -> Divide/2
  Sun Position/1 -> Length Conversion/1  "x_sun_eci"
  Clock/1 -> Divide/1
  Length Conversion/1 -> Quaternion Rotation1/2  "x_sun_eci"
  Sum1/1 -> Sun Position/1
  Radar on/off/1(Radar) -> VR Sink/8

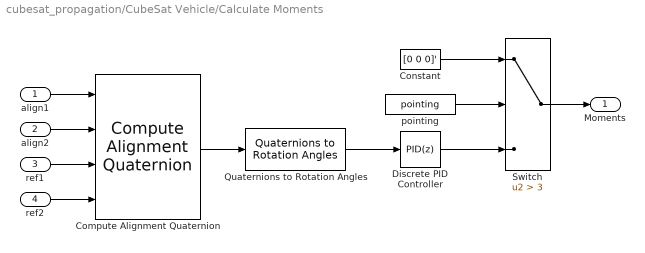
== system cubesat_propagation/CubeSat Vehicle/Calculate Moments ==
  align1 : Inport
  align2 : Inport  Port=2
  ref1 : Inport  Port=3
  ref2 : Inport  Port=4
  Compute Alignment Quaternion : asbCubeSatBlockLib/Axes Transformations/Attitude Conversion/Compute Alignment Quaternion  SystemSampleTime=-1  Latency=0  AutoFrameSizeCalculation=off
      settings: SourceProductName=Aerospace Blockset CubeSat Simulation Library  SourceProductBaseCode=AERO_CUBESAT
  Constant : Constant  Value=[0 0 0]'  OutDataTypeStr=Inherit: Inherit via back propagation
  Discrete PID Controller : simulink/Continuous/PID Controller  Controller=PID  Form=Parallel  TimeDomain=Discrete-time  SampleTime=-1  IntegratorMethod=Forward Euler  FilterMethod=Forward Euler  ControllerParametersSource=internal  P=0.00001  I=0.0000000001  D=.01  UseFilter=off  N=1000  TunerSelectOption=Transfer Function Based (PID Tuner App)  InitialConditionSource=internal  InitialConditionForIntegrator=0  InitialConditionForFilter=0  DifferentiatorICPrevScaledInput=0  ExternalReset=none  TrackingMode=off  Kt=1  LimitOutput=off  UpperSaturationLimit=inf  LowerSaturationLimit=-inf  LinearizeAsGain=off  AntiWindupMode=none  Kb=1  POutMin=[]  POutMax=[]  IOutMin=[]  IOutMax=[]  DOutMin=[]  DOutMax=[]  NOutMin=[]  NOutMax=[]  SumOutMin=[]  SumOutMax=[]  SaturationOutMin=[]  SaturationOutMax=[]  PParamMin=[]  PParamMax=[]  IParamMin=[]  IParamMax=[]  DParamMin=[]  DParamMax=[]  NParamMin=[]  NParamMax=[]  KbParamMin=[]  KbParamMax=[]  KtParamMin=[]  KtParamMax=[]  KbOutMin=[]  KbOutMax=[]  KtOutMin=[]  KtOutMax=[]  IntegratorOutMin=[]  IntegratorOutMax=[]  FilterOutMin=[]  FilterOutMax=[]  SumI1OutMin=[]  SumI1OutMax=[]  SumI2OutMin=[]  SumI2OutMax=[]  SumI3OutMin=[]  SumI3OutMax=[]  SumI4OutMin=[]  SumI4OutMax=[]  SumDOutMin=[]  SumDOutMax=[]  DifferentiatorOutMin=[]  DifferentiatorOutMax=[]  FilterDiffOutCoefMin=[]  FilterDiffOutCoefMax=[]  ReciprocalOutMin=[]  ReciprocalOutMax=[]  SumDenOutMin=[]  SumDenOutMax=[]  SumNumOutMin=[]  SumNumOutMax=[]  DivideOutMin=[]  DivideOutMax=[]  IntegratorContinuousStateAttributes=''  IntegratorStateMustResolveToSignalObject=off  IntegratorRTWStateStorageClass=Auto  FilterContinuousStateAttributes=''  FilterStateMustResolveToSignalObject=off  FilterRTWStateStorageClass=Auto  ParallelPVariant=InternalParameters  IdealPVariant=Disabled  IVariant=InternalParameters  DVariant=InternalParameters  IntegratorVariant=Discrete  SatVariant=Disabled  AWVariant=Passthrough  PCopyVariant=Disabled  TRVariant=Disabled  FdbkBlocksVariant=Forward  IdealPFdbkVariant=Disabled  SatFdbkVariant=Disabled  DerivativeFilterVariant=Differentiator  NVariant=Passthrough  NCopyVariant=Disabled_SignalSpec  FilterICVariant=InternalICsDifferentiator  IntegratorICVariant=InternalICs  ExternalResetVariant=Disabled  TRSumVariant=Passthrough  SumFdbkVariant=Disabled  SumVariant=Sum_PID
  Quaternions to Rotation Angles : sharedtransform/Quaternions to Rotation Angles  rotationOrder=XYZ  aMode=aMode
      settings: SourceProductBaseCode=AE
  Switch : Switch  Criteria=u2 > Threshold  Threshold=3
  pointing : Constant  Value=pointing  OutDataTypeStr=Inherit: Inherit via back propagation
  Moments : Outport  VectorParamsAs1DForOutWhenUnconnected=off
  wires:
  Switch/1 -> Moments/1
  Constant/1 -> Switch/1
  pointing/1 -> Switch/2
  Discrete PID Controller/1 -> Switch/3
  ref2/1 -> Compute Alignment Quaternion/4
  Compute Alignment Quaternion/1 -> Quaternions to Rotation Angles/1
  align2/1 -> Compute Alignment Quaternion/2
  ref1/1 -> Compute Alignment Quaternion/3
  align1/1 -> Compute Alignment Quaternion/1
  Quaternions to Rotation Angles/1 -> Discrete PID Controller/1

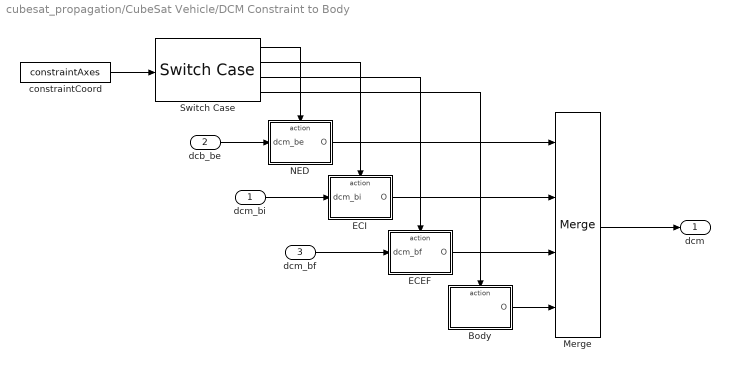
== system cubesat_propagation/CubeSat Vehicle/DCM Constraint to Body ==
  dcm_bi : Inport
  dcb_be : Inport  Port=2
  dcm_bf : Inport  Port=3
  Body : Subsystem  TreatAsAtomicUnit=on
  ECEF : Subsystem  TreatAsAtomicUnit=on
  ECI : Subsystem  TreatAsAtomicUnit=on
  Merge : Merge  Inputs=4
  NED : Subsystem  TreatAsAtomicUnit=on
  Switch Case : SwitchCase  CaseConditions={1, 2, 3, 4}  ShowDefaultCase=off
  constraintCoord : Constant  Value=constraintAxes  OutDataTypeStr=Inherit: Inherit via back propagation
  dcm : Outport  VectorParamsAs1DForOutWhenUnconnected=off
  wires:
  Merge/1 -> dcm/1
  NED/1(O) -> Merge/1
  ECI/1(O) -> Merge/2
  ECEF/1(O) -> Merge/3
  Body/1(O) -> Merge/4
  Switch Case/4 -> Body/Action
  Switch Case/3 -> ECEF/Action
  Switch Case/2 -> ECI/Action
  Switch Case/1 -> NED/Action
  dcm_bi/1 -> ECI/1(dcm_bi)
  dcm_bf/1 -> ECEF/1(dcm_bf)
  constraintCoord/1 -> Switch Case/1
  dcb_be/1 -> NED/1(dcm_be)

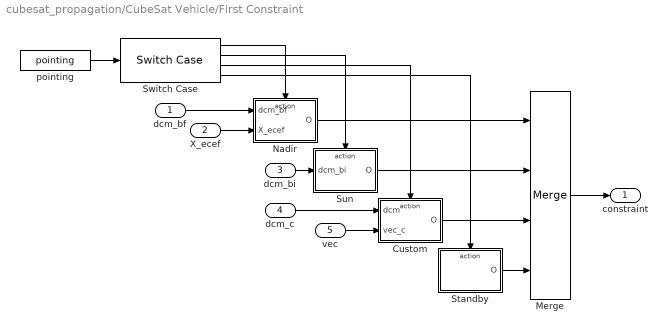
== system cubesat_propagation/CubeSat Vehicle/First Constraint ==
  dcm_bf : Inport
  X_ecef : Inport  Port=2
  dcm_bi : Inport  Port=3
  dcm_c : Inport  Port=4
  vec : Inport  Port=5
  Custom : Subsystem  TreatAsAtomicUnit=on
  Merge : Merge  Inputs=4
  Nadir : Subsystem  TreatAsAtomicUnit=on
  Standby : Subsystem  TreatAsAtomicUnit=on
  "Sun " : Subsystem  TreatAsAtomicUnit=on
  Switch Case : SwitchCase  CaseConditions={1, 2, 3}
  pointing : Constant  Value=pointing  OutDataTypeStr=Inherit: Inherit via back propagation
  constraint : Outport  VectorParamsAs1DForOutWhenUnconnected=off
  wires:
  Standby/1(O) -> Merge/4
  Switch Case/4 -> Standby/Action
  Switch Case/3 -> Custom/Action
  vec/1 -> Custom/2(vec_c)
  X_ecef/1 -> Nadir/2(X_ecef)
  dcm_bf/1 -> Nadir/1(dcm_bf)
  Merge/1 -> constraint/1
  Custom/1(O) -> Merge/3
  "Sun "/1(O) -> Merge/2
  dcm_bi/1 -> "Sun "/1(dcm_bi)
  Switch Case/1 -> Nadir/Action
  Nadir/1(O) -> Merge/1
  dcm_c/1 -> Custom/1(dcm)
  pointing/1 -> Switch Case/1
  Switch Case/2 -> "Sun "/Action

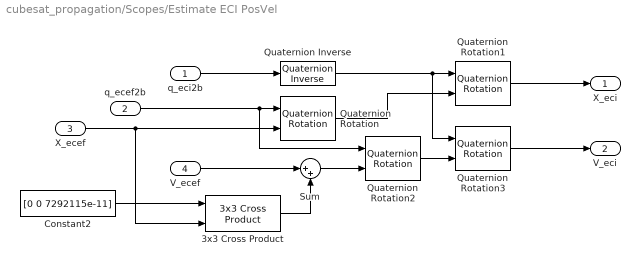
== system cubesat_propagation/Scopes/Estimate ECI PosVel ==
  q_eci2b : Inport
  q_ecef2b : Inport  Port=2
  X_ecef : Inport  Port=3
  V_ecef : Inport  Port=4
  3x3 Cross Product : sharedutil/3x3 Cross Product  aMode=aMode
      settings: SourceProductBaseCode=AE
  Constant2 : Constant  RequirementInfo={} %GIDa_da6f05bc_109e_47e8_91b9_dd401b5779d7  Value=[0 0 7292115e-11]
  Quaternion Inverse : aerolibutil/Quaternion Inverse
      settings: SourceProductName=Aerospace Blockset
  Quaternion Rotation{,1..3} (4 alike) : aerolibutil/Quaternion Rotation
  Sum : Sum  Inputs=|++
  X_eci : Outport  VectorParamsAs1DForOutWhenUnconnected=off
  V_eci : Outport  Port=2  VectorParamsAs1DForOutWhenUnconnected=off
  wires:
  Quaternion Rotation3/1 -> V_eci/1
  X_ecef/1 -> Quaternion Rotation/2, 3x3 Cross Product/2
  Quaternion Rotation1/1 -> X_eci/1
  q_eci2b/1 -> Quaternion Inverse/1
  Quaternion Rotation2/1 -> Quaternion Rotation3/2
  Constant2/1 -> 3x3 Cross Product/1
  Quaternion Inverse/1 -> Quaternion Rotation1/1, Quaternion Rotation3/1
  q_ecef2b/1 -> Quaternion Rotation2/1, Quaternion Rotation/1
  Quaternion Rotation/1 -> Quaternion Rotation1/2
  V_ecef/1 -> Sum/1
  3x3 Cross Product/1 -> Sum/2
  Sum/1 -> Quaternion Rotation2/2

== system cubesat_propagation/Scopes/Subsystem ==
  m : Inport  Unit=m
  Unit Conversion : UnitConversion
  km : Outport  Unit=km  VectorParamsAs1DForOutWhenUnconnected=off
  wires:
  Unit Conversion/1 -> km/1
  m/1 -> Unit Conversion/1

== system cubesat_propagation/Scopes/Subsystem1 ==
  m : Inport  Unit=m
  Unit Conversion : UnitConversion
  km : Outport  Unit=km  VectorParamsAs1DForOutWhenUnconnected=off
  wires:
  m/1 -> Unit Conversion/1
  Unit Conversion/1 -> km/1

== system cubesat_propagation/Scopes/Subsystem2 ==
  m/s : Inport  Unit=m/s
  Unit Conversion : UnitConversion
  km/s : Outport  Unit=km/s  VectorParamsAs1DForOutWhenUnconnected=off
  wires:
  Unit Conversion/1 -> km/s/1
  m/s/1 -> Unit Conversion/1

== system cubesat_propagation/Scopes/Subsystem3 ==
  m : Inport  Unit=m
  Unit Conversion : UnitConversion
  km : Outport  Unit=km  VectorParamsAs1DForOutWhenUnconnected=off
  wires:
  m/1 -> Unit Conversion/1
  Unit Conversion/1 -> km/1

== system cubesat_propagation/Scopes/Subsystem4 ==
  m/s : Inport  Unit=m/s
  Unit Conversion : UnitConversion
  km/s : Outport  Unit=km/s  VectorParamsAs1DForOutWhenUnconnected=off
  wires:
  Unit Conversion/1 -> km/s/1
  m/s/1 -> Unit Conversion/1

== system cubesat_propagation/Simulink 3D Animation/Antenna Position to VRML ==
  x : Inport
  ECEF to VRML : Subsystem
  Length Conversion : aerolibconvert2/Length Conversion  IU=m  OU=km
  km to VRML units : Gain  Gain=1/1000
  xVRML : Outport  VectorParamsAs1DForOutWhenUnconnected=off
  wires:
  Length Conversion/1 -> km to VRML units/1
  km to VRML units/1 -> ECEF to VRML/1(M)
  x/1 -> Length Conversion/1
  ECEF to VRML/1(VR) -> xVRML/1

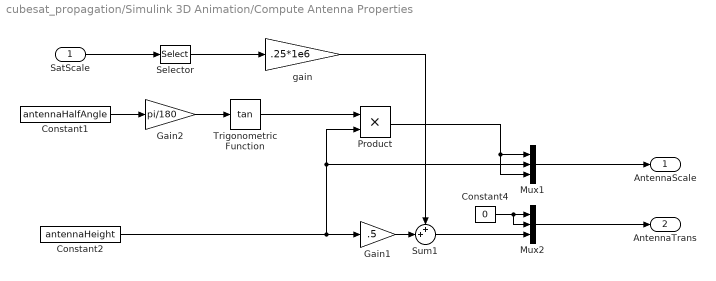
== system cubesat_propagation/Simulink 3D Animation/Compute Antenna Properties ==
  SatScale : Inport
  Constant1 : Constant  Value=antennaHalfAngle
  Constant2 : Constant  Value=antennaHeight
  Constant4 : Constant  Value=0
  Gain1 : Gain  Gain=.5
  Gain2 : Gain  Gain=pi/180
  Mux1 : Mux  Inputs=3
  Mux2 : Mux  Inputs=3
  Product : Product
  Selector : Selector  InputPortWidth=3  IndexOptions=Index vector (dialog)  Indices=1  OutputSizes=1
  Sum1 : Sum  Inputs=++|
  Trigonometric Function : Trigonometry  Operator=tan
  gain : Gain  Gain=.25*1e6
  AntennaScale : Outport  VectorParamsAs1DForOutWhenUnconnected=off
  AntennaTrans : Outport  Port=2  VectorParamsAs1DForOutWhenUnconnected=off
  wires:
  Gain2/1 -> Trigonometric Function/1
  Constant4/1 -> Mux2/1, Mux2/2
  Sum1/1 -> Mux2/3
  Constant2/1 -> Gain1/1, Mux1/2, Product/2
  gain/1 -> Sum1/1
  Constant1/1 -> Gain2/1
  Product/1 -> Mux1/3, Mux1/1
  Gain1/1 -> Sum1/2
  Trigonometric Function/1 -> Product/1
  Mux2/1 -> AntennaTrans/1
  Mux1/1 -> AntennaScale/1
  SatScale/1 -> Selector/1
  Selector/1 -> gain/1

== system cubesat_propagation/Simulink 3D Animation/Compute Earth Rotation Rate ==
  EarthRot : Inport
  Constant : Constant  Value=0
  Constant1 : Constant  Value=0
  Euler Angles to Quaternions : aerolibobsolete/Euler Angles to Quaternions
      settings: SourceProductName=Aerospace Blockset  SourceProductBaseCode=AE
  Quaternion to VRML : Subsystem
  Sum : Sum  Inputs=|++
  Unit Delay : UnitDelay  SampleTime=-1  HasFrameUpgradeWarning=on
  Vector Concatenate : Concatenate  NumInputs=3
  VRMLRot : Outport  VectorParamsAs1DForOutWhenUnconnected=off
  wires:
  Quaternion to VRML/1(AxisAngle) -> VRMLRot/1
  Euler Angles to Quaternions/1 -> Quaternion to VRML/1(q)
  Vector Concatenate/1 -> Euler Angles to Quaternions/1
  Constant1/1 -> Vector Concatenate/2
  Constant/1 -> Vector Concatenate/1
  Sum/1 -> Unit Delay/1, Vector Concatenate/3
  Unit Delay/1 -> Sum/2
  EarthRot/1 -> Sum/1

== system cubesat_propagation/Simulink 3D Animation/Compute Umbra Translation ==
  I : Inport
  Add : Sum
  ConeHalfLength : Gain  Gain=692
  InvertSunPosECEF : Gain  Gain=-1
  unitVec : Subsystem
  O : Outport  VectorParamsAs1DForOutWhenUnconnected=off
  wires:
  ConeHalfLength/1 -> Add/2
  I/1 -> InvertSunPosECEF/1
  Add/1 -> O/1
  InvertSunPosECEF/1 -> unitVec/1(I), Add/1
  unitVec/1(O) -> ConeHalfLength/1

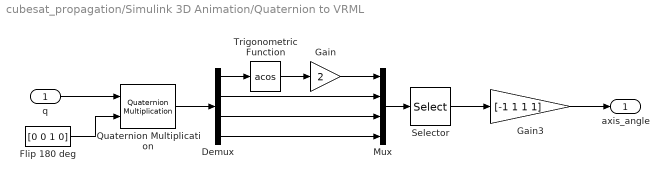
== system cubesat_propagation/Simulink 3D Animation/Quaternion to VRML ==
  q : Inport
  Demux : Demux
  Flip 180 deg : Constant  Value=[0 0 1 0]
  Gain : Gain  Gain=2
  Gain3 : Gain  Gain=[-1 1 1 1]
  Mux : Mux
  Quaternion Multiplication : aerolibutil/Quaternion Multiplication
  Selector : Selector  InputPortWidth=4  IndexOptions=Index vector (dialog)  Indices=[2 4 3 1]  OutputSizes=1
  Trigonometric Function : Trigonometry  Operator=acos
  axis_angle : Outport  VectorParamsAs1DForOutWhenUnconnected=off
  wires:
  Demux/4 -> Mux/4
  Demux/3 -> Mux/3
  Demux/2 -> Mux/2
  Gain/1 -> Mux/1
  Selector/1 -> Gain3/1
  Gain3/1 -> axis_angle/1
  q/1 -> Quaternion Multiplication/1
  Mux/1 -> Selector/1
  Trigonometric Function/1 -> Gain/1
  Demux/1 -> Trigonometric Function/1
  Flip 180 deg/1 -> Quaternion Multiplication/2
  Quaternion Multiplication/1 -> Demux/1

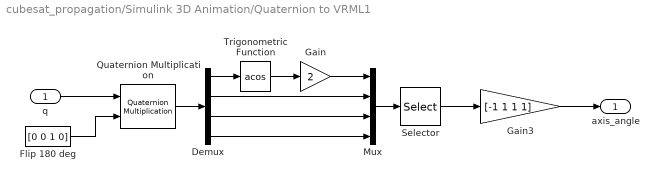
== system cubesat_propagation/Simulink 3D Animation/Quaternion to VRML1 ==
  q : Inport
  Demux : Demux
  Flip 180 deg : Constant  Value=[0 0 1 0]
  Gain : Gain  Gain=2
  Gain3 : Gain  Gain=[-1 1 1 1]
  Mux : Mux
  Quaternion Multiplication : aerolibutil/Quaternion Multiplication
  Selector : Selector  InputPortWidth=4  IndexOptions=Index vector (dialog)  Indices=[2 4 3 1]  OutputSizes=1
  Trigonometric Function : Trigonometry  Operator=acos
  axis_angle : Outport  VectorParamsAs1DForOutWhenUnconnected=off
  wires:
  Demux/4 -> Mux/4
  Demux/3 -> Mux/3
  Demux/2 -> Mux/2
  Gain/1 -> Mux/1
  Selector/1 -> Gain3/1
  Gain3/1 -> axis_angle/1
  Mux/1 -> Selector/1
  Trigonometric Function/1 -> Gain/1
  Demux/1 -> Trigonometric Function/1
  Flip 180 deg/1 -> Quaternion Multiplication/2
  q/1 -> Quaternion Multiplication/1
  Quaternion Multiplication/1 -> Demux/1

== system cubesat_propagation/Simulink 3D Animation/Radar on//off ==
  NavMode : Inport
  Add : Sum  Inputs=-+
  Compare To Constant : simulink/Logic and Bit Operations/Compare To Constant  relop===  const=1  OutDataTypeStr=boolean  ZeroCross=off
  Constant : Constant
  Data Type Conversion : DataTypeConversion  OutDataTypeStr=double
  Gain : Gain  Gain=0.6
  Radar : Outport  VectorParamsAs1DForOutWhenUnconnected=off
  wires:
  NavMode/1 -> Compare To Constant/1
  Compare To Constant/1 -> Data Type Conversion/1
  Data Type Conversion/1 -> Gain/1
  Gain/1 -> Add/1
  Constant/1 -> Add/2
  Add/1 -> Radar/1

== system cubesat_propagation/Simulink 3D Animation/Sat Position to VRML ==
  x : Inport
  ECEF to VRML : Subsystem
  Length Conversion : aerolibconvert2/Length Conversion  IU=m  OU=km
  km to VRML units : Gain  Gain=1/1000
  xVRML : Outport  VectorParamsAs1DForOutWhenUnconnected=off
  wires:
  ECEF to VRML/1(VR) -> xVRML/1
  x/1 -> Length Conversion/1
  km to VRML units/1 -> ECEF to VRML/1(M)
  Length Conversion/1 -> km to VRML units/1

== system cubesat_propagation/Simulink 3D Animation/Satellite Model Scaling ==
  Constant : Constant  Value=cubesatSize
  Mux : Mux  Inputs=3
  ScaleModelToVRML : Gain  Gain=1/.3e6
  Out1 : Outport  VectorParamsAs1DForOutWhenUnconnected=off
  wires:
  ScaleModelToVRML/1 -> Mux/3, Mux/1, Mux/2
  Constant/1 -> ScaleModelToVRML/1
  Mux/1 -> Out1/1

== system cubesat_propagation/Simulink 3D Animation/Sun Position to VRML ==
  x : Inport
  ECEF to VRML : Subsystem
  Length Conversion : aerolibconvert2/Length Conversion  IU=m  OU=km
  km to VRML units : Gain  Gain=1/1000
  xVRML : Outport  VectorParamsAs1DForOutWhenUnconnected=off
  wires:
  ECEF to VRML/1(VR) -> xVRML/1
  x/1 -> Length Conversion/1
  km to VRML units/1 -> ECEF to VRML/1(M)
  Length Conversion/1 -> km to VRML units/1

== system cubesat_propagation/CubeSat Vehicle/DCM Constraint to Body/Body ==
  Action Port : ActionPort  ActionPortLabel=case [ 4 ]:
  Constant : Constant  Value=eye(3)
  O : Outport  VectorParamsAs1DForOutWhenUnconnected=off
  wires:
  Constant/1 -> O/1

== system cubesat_propagation/CubeSat Vehicle/DCM Constraint to Body/ECEF ==
  dcm_bf : Inport
  Action Port : ActionPort  ActionPortLabel=case [ 3 ]:
  O : Outport  VectorParamsAs1DForOutWhenUnconnected=off
  wires:
  dcm_bf/1 -> O/1

== system cubesat_propagation/CubeSat Vehicle/DCM Constraint to Body/ECI ==
  dcm_bi : Inport
  Action Port : ActionPort  ActionPortLabel=case [ 2 ]:
  O : Outport  VectorParamsAs1DForOutWhenUnconnected=off
  wires:
  dcm_bi/1 -> O/1

== system cubesat_propagation/CubeSat Vehicle/DCM Constraint to Body/NED ==
  dcm_be : Inport
  Action Port : ActionPort  ActionPortLabel=case [ 1 ]:
  O : Outport  VectorParamsAs1DForOutWhenUnconnected=off
  wires:
  dcm_be/1 -> O/1

== system cubesat_propagation/CubeSat Vehicle/First Constraint/Custom ==
  dcm : Inport
  vec_c : Inport  Port=2
  Action Port : ActionPort  ActionPortLabel=case [ 3 ]:
  Matrix Multiply : Product  Multiplication=Matrix(*)
  Reshape3 : Reshape
  O : Outport  VectorParamsAs1DForOutWhenUnconnected=off
  wires:
  Matrix Multiply/1 -> O/1
  Reshape3/1 -> Matrix Multiply/2
  dcm/1 -> Matrix Multiply/1
  vec_c/1 -> Reshape3/1

== system cubesat_propagation/CubeSat Vehicle/First Constraint/Nadir ==
  dcm_bf : Inport
  X_ecef : Inport  Port=2
  Action Port : ActionPort  ActionPortLabel=case [ 1 ]:
  Gain : Gain  Gain=-1
  Matrix Multiply : Product  Multiplication=Matrix(*)
  O : Outport  VectorParamsAs1DForOutWhenUnconnected=off
  wires:
  Matrix Multiply/1 -> O/1
  Gain/1 -> Matrix Multiply/2
  X_ecef/1 -> Gain/1
  dcm_bf/1 -> Matrix Multiply/1

== system cubesat_propagation/CubeSat Vehicle/First Constraint/Standby ==
  Action Port : ActionPort  ActionPortLabel=default:
  Constant : Constant  Value=[0 0 0]'  OutDataTypeStr=Inherit: Inherit via back propagation
  O : Outport  VectorParamsAs1DForOutWhenUnconnected=off
  wires:
  Constant/1 -> O/1

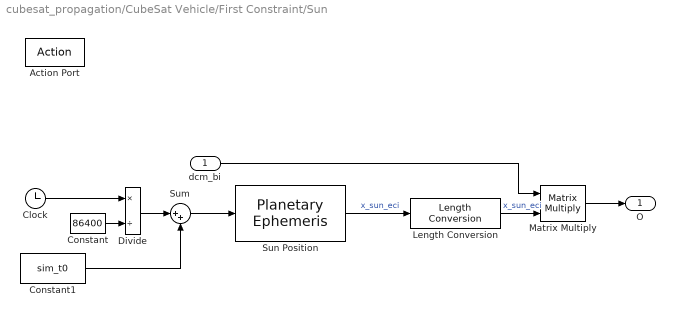
== system cubesat_propagation/CubeSat Vehicle/First Constraint/Sun  ==
  dcm_bi : Inport
  Action Port : ActionPort  ActionPortLabel=case [ 2 ]:
  Clock : Clock
  Constant : Constant  Value=86400
  Constant1 : Constant  RequirementInfo={} %GIDa_3340d8fb_5b7e_4e83_88e1_92a85cc7add9  Value=sim_t0
  Divide : Product  Inputs=*/
  Length Conversion : aerolibconvert2/Length Conversion  IU=km  OU=m
  Matrix Multiply : Product  Multiplication=Matrix(*)
  Sum : Sum  Inputs=|++
  Sun Position : aerolibcelestial/Planetary Ephemeris  kmflag=km,km/s  epochflag=Julian date  de=DE421  nCenter=Earth  nTarget=Sun  errorflag=Error  velflag=off
      settings: SourceProductName=Aerospace Blockset  SourceProductBaseCode=AE
  O : Outport  VectorParamsAs1DForOutWhenUnconnected=off
  wires:
  Matrix Multiply/1 -> O/1
  Length Conversion/1 -> Matrix Multiply/2  "x_sun_eci"
  Divide/1 -> Sum/1
  Constant/1 -> Divide/2
  Sun Position/1 -> Length Conversion/1  "x_sun_eci"
  Clock/1 -> Divide/1
  Sum/1 -> Sun Position/1
  Constant1/1 -> Sum/2
  dcm_bi/1 -> Matrix Multiply/1

== system cubesat_propagation/Simulink 3D Animation/Antenna Position to VRML/ECEF to VRML ==
  M : Inport  PortDimensions=3
  Demux : Demux  Outputs=3
  Gain3 : Gain  Gain=-1
  Mux : Mux  Inputs=3
  VR : Outport  PortDimensions=3  VectorParamsAs1DForOutWhenUnconnected=off
  wires:
  M/1 -> Demux/1
  Demux/1 -> Gain3/1
  Demux/2 -> Mux/3
  Demux/3 -> Mux/2
  Mux/1 -> VR/1
  Gain3/1 -> Mux/1
